simulink model "ANN_based_PI_Controlled_SAPF_pq_theory"  (R2023b)
settings: Solver=ode45  StartTime=0.0  StopTime=5  RelTol=1e-3  EnableMultiTasking=on
model workspace (MAT data in the model file):
  Ki = 1
  Kp = 0.1
libraries: spsDiodeLib x6, spsSeriesRLCBranchLib x5, spsCurrentMeasurementLib x4, spsThreePhaseBreakerLib x3, spsThreePhaseVIMeasurementLib x3, spsVoltageMeasurementLib x2, spsThreePhaseSeriesRLCBranchLib x2, spsThreePhaseSourceLib x1, simulink x1, dspfdesign x1, spsUniversalBridgeLib x1, sps_lib x1
settings Model: Creator=Jawad  LastModifiedBy=khana
settings SolverCC: AlgebraicLoopSolver=TrustRegion
settings DataIOCC: LimitDataPoints=on  SaveFormat=Array  SignalLoggingSaveFormat=ModelDataLogs  ReturnWorkspaceOutputs=off
settings OptimizationCC: ExpressionDepthLimit=2147483647  LifeSpan=inf
settings DebuggingCC: UnderspecifiedInitializationDetection=Classic  MergeDetectMultiDrivingBlocksExec=none  SolverPrmCheckMsg=warning  FcnCallInpInsideContextMsg=warning  UnconnectedInputMsg=warning  UnconnectedOutputMsg=warning  UnconnectedLineMsg=warning  StateNameClashWarn=warning  SFUnexpectedBacktrackingDiag=warning  SFNoUnconditionalDefaultTransitionDiag=warning  SFExecutionAtInitializationDiag=none  ArithmeticOperatorsInVariantConditions=warning
settings HardwareCC: ProdBitPerPointer=32  ProdBitPerSizeT=32  ProdBitPerPtrDiffT=32  ProdLargestAtomicFloat=None  ProdIntDivRoundTo=Undefined  ProdEndianess=Unspecified  ProdWordSize=32  ProdHWDeviceType=32-bit Generic
settings ModelReferenceCC: PropagateSignalLabelsOutOfModel=off
settings SFSimCC: SimUseLocalCustomCode=off  SimParseCustomCode=off  CustomCodeUndefinedFunction=UseInterfaceOnly
settings RTWCC: RTWUseLocalCustomCode=off
settings CodeAppCC: StateflowObjectComments=on
settings GRTTargetCC: TargetLangStandard=C89/C90 (ANSI)  CombineOutputUpdateFcns=off  GRTInterface=on
settings ConfigComp: CovMetricSettings=dw  CovSaveCumulativeToWorkspaceVar=on  CovSaveSingleToWorkspaceVar=on  CovExternalEMLEnable=off

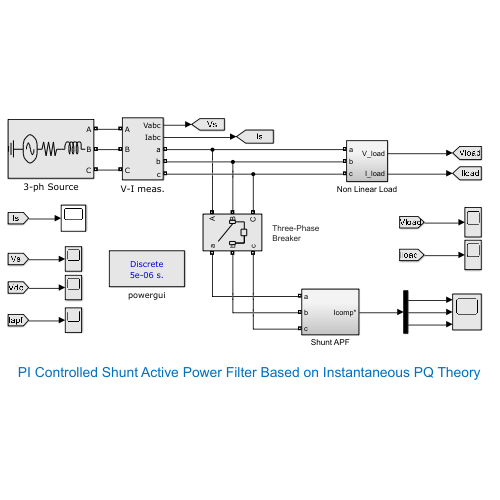
[thumbnail: Simulink's stored preview of the top-level diagram]
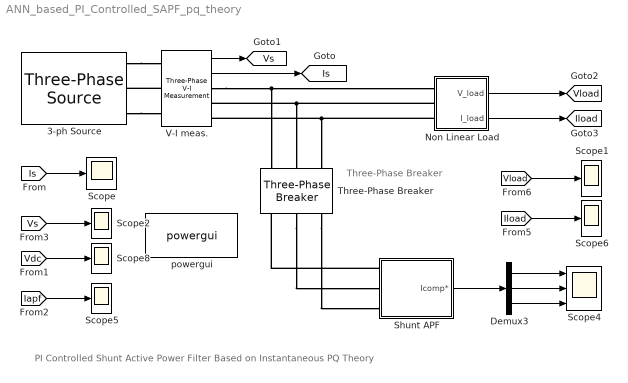
== system ANN_based_PI_Controlled_SAPF_pq_theory ==
  note: Three-Phase Breaker
  note: PI Controlled Shunt Active Power Filter Based on Instantaneous PQ Theory
  3-ph Source : spsThreePhaseSourceLib/Three-Phase Source  InternalConnection=Yg  VoltagePhases=off  Voltage=40  PhaseAngle=0  Voltage_phases=[25e3 25e3 25e3]/sqrt(3)  PhaseAngles_phases=[0 -120 +120]  Frequency=50  NonIdealSource=on  SpecifyImpedance=off  Resistance=0.001  Inductance=1e-8  ShortCircuitLevel=100e6  BaseVoltage=25e3  XRratio=7  BusType=swing  Pref=10e3  Qref=0  Prefabc=[10e3, 10e3, 10e3]  Qrefabc=[0, 0, 0]  Qmin=-inf  Qmax=inf
  Demux3 : Demux  Outputs=3
  Non Linear Load : Subsystem
  Scope{,1..2,5..6,8} (6 alike) : Scope
  Scope4 : Scope  NumInputPorts=3
  Shunt APF : Subsystem
  Three-Phase Breaker : spsThreePhaseBreakerLib/Three-Phase Breaker  InitialState=open  SwitchA=on  SwitchB=on  SwitchC=on  SwitchTimes=0.02  External=off  BreakerResistance=1e-6  SnubberResistance=1e6  SnubberCapacitance=inf  Measurements=None
  V-I meas. : spsThreePhaseVIMeasurementLib/Three-Phase V-I Measurement  VoltageMeasurement=phase-to-ground  SetLabelV=off  LabelV=Vabc  Vpu=off  VpuLL=off  CurrentMeasurement=yes  SetLabelI=off  LabelI=Iabc  Ipu=off  Pbase=100e6  Vbase=500e3  OutputType=Complex  PhasorSimulation=off  PSBequivalent=0
  powergui : sps_lib/powergui  Priority=1  SimulationMode=Discrete  SampleTime=5e-6  frequency=60  Iterations=50  frequencyindice=50  Pbase=100e6  ErrMax=1e-4  UnitsV=kV  UnitsW=MW  buscounter=0  FunctionMessages=off  echomessages=off  EnableUseOfTLC=off  CurrentSourceSwitches=off  DisableSnubberDevices=off  DisableRonSwitches=off  DisableVfSwitches=off  DisplayEquations=off  AutomaticDiscreteSolvers=off  SolverType=Tustin/Backward Euler (TBE)  Interpol=off  ExternalGateDelay=off  methode=off  Ts=100  x0status=blocks  SPID=off  SwTol=0  HookPort=off  NonlinearTolerance=1e-4  nMaxIteration=100  ContinueOnMaxIteration=off  RestoreLinks=warning  ResistiveCurrentMeasurement=off  Frange=[0:2:500]  Ylog=off  Xlog=on  ShowGrid=off  save=off  variable=ZData  structure=psb3phPWM1_str8  ZoomFFT=off  StartTime=0.035  cycles=2  DisplayStyle=2  fundamental=50  FreqAxis=off  MaxFrequency=10000  frequencyindicesteady=1  RmsSteady=1  display=off
  tag scope: Iload=global, Is=global, Vload=global, Vs=global
  wires:
  Non Linear Load/2(I_load) -> [Iload]
  V-I meas./1 -> [Vs]
  V-I meas./2 -> [Is]
  Demux3/1 -> Scope4/1
  Demux3/2 -> Scope4/2
  Demux3/3 -> Scope4/3
  Shunt APF/1(Icomp*) -> Demux3/1
  [Is] -> Scope/1
  [Vs] -> Scope2/1
  [Vdc] -> Scope8/1
  [Iapf] -> Scope5/1
  [Vload] -> Scope1/1
  [Iload] -> Scope6/1
  Non Linear Load/1(V_load) -> [Vload]
  connections:
  3-ph Source/RConn1 -- V-I meas./LConn1
  V-I meas./LConn2 -- 3-ph Source/RConn2
  3-ph Source/RConn3 -- V-I meas./LConn3
  V-I meas./RConn1 -- Three-Phase Breaker/LConn1 -- Non Linear Load/LConn1
  Non Linear Load/LConn2 -- Three-Phase Breaker/LConn2 -- V-I meas./RConn2
  Non Linear Load/LConn3 -- Three-Phase Breaker/LConn3 -- V-I meas./RConn3
  Shunt APF/LConn1 -- Three-Phase Breaker/RConn1
  Three-Phase Breaker/RConn2 -- Shunt APF/LConn2
  Three-Phase Breaker/RConn3 -- Shunt APF/LConn3

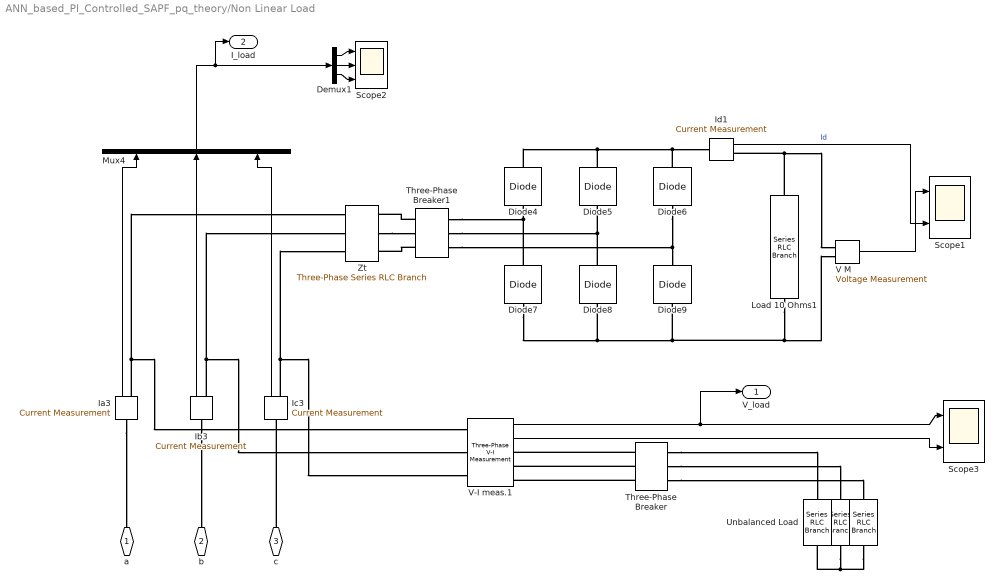
== system ANN_based_PI_Controlled_SAPF_pq_theory/Non Linear Load ==
  " " : spsSeriesRLCBranchLib/Series RLC Branch  LConnTagsString=__new0  RConnTagsString=__new0  BranchType=R  Resistance=4  Inductance=[]  SetiL0=off  InitialCurrent=0  Capacitance=[]  Setx0=off  InitialVoltage=0  Measurements=None
  "   " : spsSeriesRLCBranchLib/Series RLC Branch  LConnTagsString=__new0  RConnTagsString=__new0  BranchType=R  Resistance=6  Inductance=[]  SetiL0=off  InitialCurrent=0  Capacitance=[]  Setx0=off  InitialVoltage=0  Measurements=None
  Demux1 : Demux  Outputs=3
  Diode{4..9} (6 alike) : spsDiodeLib/Diode  Ron=1e-1  Lon=0  Vf=0.8  IC=0  UseSnubber=off  Rs=1000  Cs=0.1e-6  Measurements=off
      settings: AttributesFormatString=\n
  Ia3 : spsCurrentMeasurementLib/Current Measurement  PhasorSimulation=off  OutputType=Complex  PSBequivalent=0
  Ib3 : spsCurrentMeasurementLib/Current Measurement  PhasorSimulation=off  OutputType=Complex  PSBequivalent=0
  Ic3 : spsCurrentMeasurementLib/Current Measurement  PhasorSimulation=off  OutputType=Complex  PSBequivalent=0
  Id1 : spsCurrentMeasurementLib/Current Measurement  Tag=PoWeRsYsTeMmEaSuReMeNt  PhasorSimulation=off  OutputType=Magnitude  PSBequivalent=0
      settings: AttributesFormatString=\n
  Load 10 Ohms1 : spsSeriesRLCBranchLib/Series RLC Branch  LConnTagsString=__new0  RConnTagsString=__new0  BranchType=RL  Resistance=60  Inductance=10e-3  SetiL0=off  InitialCurrent=0  Capacitance=[]  Setx0=off  InitialVoltage=0  Measurements=None
  Mux4 : Mux  Inputs=3
  Scope1 : Scope  NumInputPorts=2
  Scope2 : Scope  NumInputPorts=3
  Scope3 : Scope  NumInputPorts=2
  Three-Phase Breaker : spsThreePhaseBreakerLib/Three-Phase Breaker  InitialState=open  SwitchA=on  SwitchB=on  SwitchC=on  SwitchTimes=0.2  External=off  BreakerResistance=1e-5  SnubberResistance=1e6  SnubberCapacitance=inf  Measurements=None
  Three-Phase Breaker1 : spsThreePhaseBreakerLib/Three-Phase Breaker  InitialState=open  SwitchA=on  SwitchB=on  SwitchC=on  SwitchTimes=0  External=off  BreakerResistance=1e-5  SnubberResistance=1e6  SnubberCapacitance=inf  Measurements=None
  Unbalanced Load : spsSeriesRLCBranchLib/Series RLC Branch  LConnTagsString=__new0  RConnTagsString=__new0  BranchType=R  Resistance=2  Inductance=[]  SetiL0=off  InitialCurrent=0  Capacitance=[]  Setx0=off  InitialVoltage=0  Measurements=None
  V M : spsVoltageMeasurementLib/Voltage Measurement  PhasorSimulation=off  OutputType=Complex  PSBequivalent=0
  V-I meas.1 : spsThreePhaseVIMeasurementLib/Three-Phase V-I Measurement  VoltageMeasurement=phase-to-ground  SetLabelV=off  LabelV=Vabc  Vpu=off  VpuLL=off  CurrentMeasurement=yes  SetLabelI=off  LabelI=Iabc  Ipu=off  Pbase=100e6  Vbase=500e3  OutputType=Complex  PhasorSimulation=off  PSBequivalent=0
  Zt : spsThreePhaseSeriesRLCBranchLib/Three-Phase Series RLC Branch  LConnTagsString=A|B|C  RConnTagsString=A|B|C  BranchType=RL  Resistance=0.01  Inductance=1e-3  Capacitance=1e-6  Measurements=None
  a : PMIOPort  Side=Left
  b : PMIOPort  Port=2  Side=Left
  c : PMIOPort  Port=3  Side=Left
  V_load : Outport
  I_load : Outport  Port=2
  wires:
  Mux4/1 -> I_load/1, Demux1/1
  Demux1/2 -> Scope2/2
  Demux1/3 -> Scope2/3
  Demux1/1 -> Scope2/1
  V M/1 -> Scope1/1
  Id1/1 -> Scope1/2  "Id"
  V-I meas.1/1 -> Scope3/1, V_load/1
  V-I meas.1/2 -> Scope3/2
  Ic3/1 -> Mux4/3
  Ib3/1 -> Mux4/2
  Ia3/1 -> Mux4/1
  connections:
  Ia3/LConn1 -- a/RConn1
  Ib3/LConn1 -- b/RConn1
  Ic3/RConn1 -- V-I meas.1/LConn3 -- Zt/LConn3
  Ib3/RConn1 -- V-I meas.1/LConn2 -- Zt/LConn2
  Ia3/RConn1 -- V-I meas.1/LConn1 -- Zt/LConn1
  Diode6/RConn1 -- Id1/LConn1 -- Diode4/RConn1 -- Diode5/RConn1
  Load 10 Ohms1/LConn1 -- Id1/RConn1 -- V M/LConn1
  Diode9/LConn1 -- Diode7/LConn1 -- Diode8/LConn1 -- V M/LConn2 -- Load 10 Ohms1/RConn1
  Unbalanced Load/RConn1 -- " "/RConn1 -- "   "/RConn1
  c/RConn1 -- Ic3/LConn1
  Three-Phase Breaker/LConn3 -- V-I meas.1/RConn3
  Three-Phase Breaker/LConn2 -- V-I meas.1/RConn2
  Three-Phase Breaker/LConn1 -- V-I meas.1/RConn1
  Three-Phase Breaker/RConn1 -- Unbalanced Load/LConn1
  Three-Phase Breaker/RConn2 -- " "/LConn1
  Three-Phase Breaker/RConn3 -- "   "/LConn1
  Diode7/RConn1 -- Three-Phase Breaker1/RConn1 -- Diode4/LConn1
  Diode8/RConn1 -- Three-Phase Breaker1/RConn2 -- Diode5/LConn1
  Diode6/LConn1 -- Diode9/RConn1 -- Three-Phase Breaker1/RConn3
  Three-Phase Breaker1/LConn1 -- Zt/RConn1
  Zt/RConn2 -- Three-Phase Breaker1/LConn2
  Three-Phase Breaker1/LConn3 -- Zt/RConn3

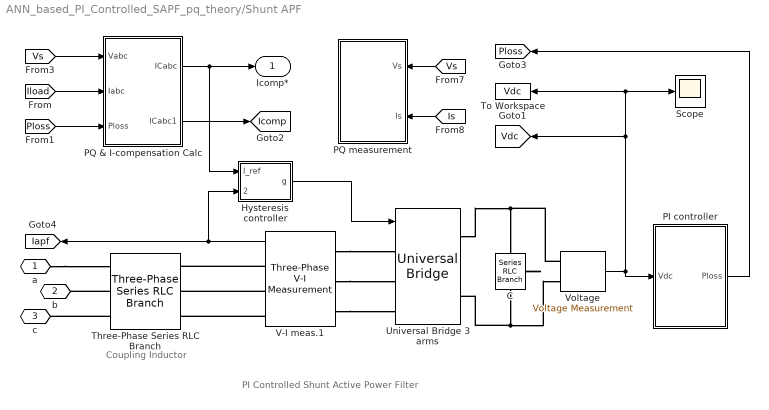
== system ANN_based_PI_Controlled_SAPF_pq_theory/Shunt APF ==
  note: Coupling Inductor
  note: PI Controlled Shunt Active Power Filter
  C : spsSeriesRLCBranchLib/Series RLC Branch  LConnTagsString=__new0  RConnTagsString=__new0  BranchType=C  Resistance=1  Inductance=1e-3  SetiL0=off  InitialCurrent=0  Capacitance=3.5e-6  Setx0=off  InitialVoltage=400  Measurements=None
  Hysteresis controller : Subsystem
  PI controller : Subsystem
  PQ & I-compensation Calc : Subsystem
  PQ measurement : Subsystem
  Scope : Scope
  Three-Phase Series RLC Branch : spsThreePhaseSeriesRLCBranchLib/Three-Phase Series RLC Branch  LConnTagsString=A|B|C  RConnTagsString=A|B|C  BranchType=L  Resistance=1e9  Inductance=10e-3  Capacitance=.2e-3  Measurements=None
  To Workspace : ToWorkspace  VariableName=Vdc  SaveFormat=Timeseries  SampleTime=-1
  Universal Bridge 3 arms : spsUniversalBridgeLib/Universal Bridge  Arms=3  SnubberResistance=10000  SnubberCapacitance=inf  Device=IGBT / Diodes  Ron=1e-4  Lon=0  ForwardVoltages="[  1  1  ]"  ForwardVoltage=.8  GTOparameters=[ 10e-6 , 20e-6 ]  IGBTparameters=[ 1e-6 , 2e-6 ]  Measurements=None  Measurements_2=None  converterType=Rectifier
      settings: AttributesFormatString=\n
  V-I meas.1 : spsThreePhaseVIMeasurementLib/Three-Phase V-I Measurement  VoltageMeasurement=phase-to-ground  SetLabelV=on  LabelV=Vnm  Vpu=off  VpuLL=off  CurrentMeasurement=yes  SetLabelI=off  LabelI=Iabc  Ipu=off  Pbase=100e6  Vbase=500e3  OutputType=Complex  PhasorSimulation=off  PSBequivalent=0
  Voltage : spsVoltageMeasurementLib/Voltage Measurement  PhasorSimulation=off  OutputType=Complex  PSBequivalent=0
  a : PMIOPort  Side=Left
  b : PMIOPort  Port=2  Side=Left
  c : PMIOPort  Port=3  Side=Left
  Icomp* : Outport
  tag scope: Iapf=global, Icomp=global, Ploss=global, Vdc=global
  wires:
  [Iload] -> PQ & I-compensation Calc/2(Iabc)
  V-I meas.1/1 -> [Iapf], Hysteresis controller/2(I_meas)
  Hysteresis controller/1(g) -> Universal Bridge 3 arms/1
  PQ & I-compensation Calc/1(ICabc) -> Icomp*/1, Hysteresis controller/1(I_ref)
  Voltage/1 -> To Workspace/1, Scope/1, [Vdc], PI controller/1(Vdc)
  [Vs] -> PQ & I-compensation Calc/1(Vabc)
  PQ & I-compensation Calc/2(ICabc1) -> [Icomp]
  PI controller/1(Ploss) -> [Ploss]
  [Ploss] -> PQ & I-compensation Calc/3(Ploss)
  [Vs] -> PQ measurement/1(Vs)
  [Is] -> PQ measurement/2(Is)
  connections:
  Voltage/LConn1 -- C/LConn1 -- Universal Bridge 3 arms/RConn1
  V-I meas.1/LConn1 -- Universal Bridge 3 arms/LConn1
  V-I meas.1/LConn2 -- Universal Bridge 3 arms/LConn2
  V-I meas.1/RConn3 -- Three-Phase Series RLC Branch/LConn3
  V-I meas.1/RConn2 -- Three-Phase Series RLC Branch/LConn2
  V-I meas.1/LConn3 -- Universal Bridge 3 arms/LConn3
  V-I meas.1/RConn1 -- Three-Phase Series RLC Branch/LConn1
  a/RConn1 -- Three-Phase Series RLC Branch/RConn1
  Three-Phase Series RLC Branch/RConn2 -- b/RConn1
  Three-Phase Series RLC Branch/RConn3 -- c/RConn1
  C/RConn1 -- Voltage/LConn2 -- Universal Bridge 3 arms/RConn2

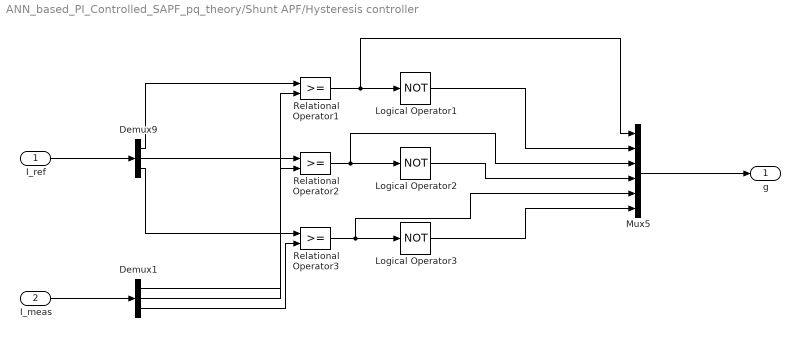
== system ANN_based_PI_Controlled_SAPF_pq_theory/Shunt APF/Hysteresis controller ==
  I_ref : Inport
  I_meas : Inport  Port=2
  Demux1 : Demux  Outputs=3
  Demux9 : Demux  Outputs=3
  Logical Operator1 : Logic  Operator=NOT  AllPortsSameDT=off  OutDataTypeStr=boolean
  Logical Operator2 : Logic  Operator=NOT  AllPortsSameDT=off  OutDataTypeStr=boolean
  Logical Operator3 : Logic  Operator=NOT  AllPortsSameDT=off  OutDataTypeStr=boolean
  Mux5 : Mux  Inputs=6
  Relational Operator1 : RelationalOperator  OutDataTypeStr=boolean  ZeroCross=off  InputSameDT=off
  Relational Operator2 : RelationalOperator  OutDataTypeStr=boolean  ZeroCross=off  InputSameDT=off
  Relational Operator3 : RelationalOperator  OutDataTypeStr=boolean  ZeroCross=off  InputSameDT=off
  g : Outport
  wires:
  Relational Operator1/1 -> Logical Operator1/1, Mux5/1
  Relational Operator2/1 -> Logical Operator2/1, Mux5/3
  Relational Operator3/1 -> Logical Operator3/1, Mux5/5
  Demux9/1 -> Relational Operator1/1
  Demux9/3 -> Relational Operator3/1
  Logical Operator1/1 -> Mux5/2
  Logical Operator2/1 -> Mux5/4
  Logical Operator3/1 -> Mux5/6
  Mux5/1 -> g/1
  Demux9/2 -> Relational Operator2/1
  Demux1/1 -> Relational Operator1/2
  Demux1/2 -> Relational Operator2/2
  Demux1/3 -> Relational Operator3/2
  I_ref/1 -> Demux9/1
  I_meas/1 -> Demux1/1

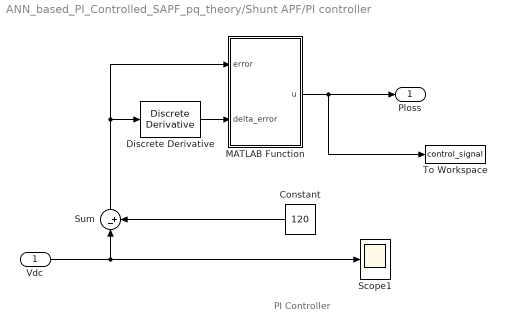
== system ANN_based_PI_Controlled_SAPF_pq_theory/Shunt APF/PI controller ==
  note: PI Controller
  Vdc : Inport
  Constant : Constant  Value=120
  Discrete Derivative : simulink/Discrete/Discrete Derivative  gainval=1.0  ICPrevScaledInput=0.0  OutMin=[]  OutMax=[]  OutDataType=fixdt(1, 16)  OutScaling=2^-10  DoSatur=off
  MATLAB Function : MATLAB Function  TreatAsAtomicUnit=on
  Scope1 : Scope
  Sum : Sum  Inputs=|-+
  To Workspace : ToWorkspace  VariableName=control_signal  SaveFormat=Timeseries  SampleTime=-1
  Ploss : Outport
  wires:
  Constant/1 -> Sum/2
  Sum/1 -> MATLAB Function/1(error), Discrete Derivative/1
  MATLAB Function/1(u) -> Ploss/1, To Workspace/1
  Vdc/1 -> Scope1/1, Sum/1
  Discrete Derivative/1 -> MATLAB Function/2(delta_error)

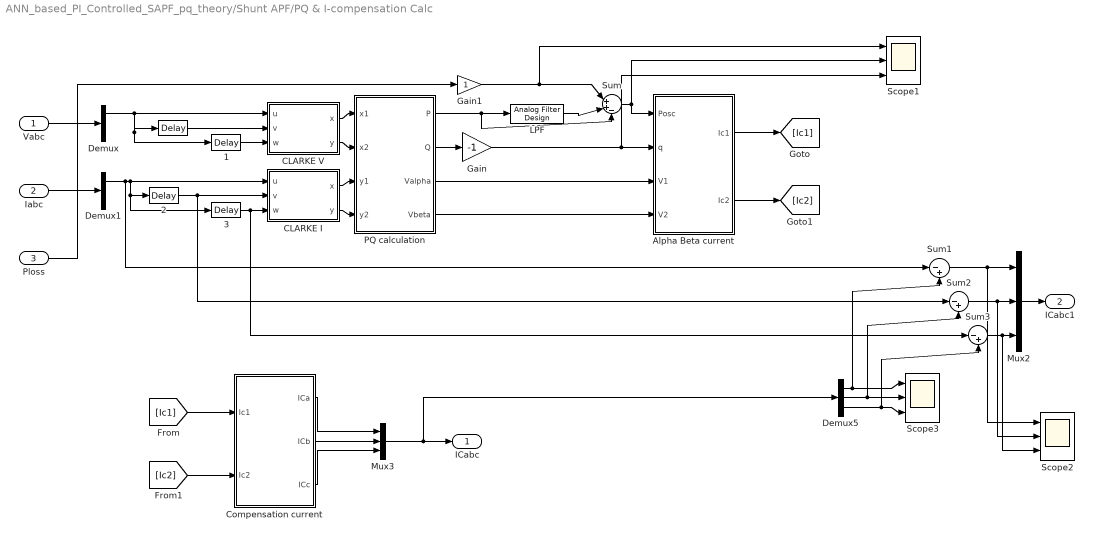
== system ANN_based_PI_Controlled_SAPF_pq_theory/Shunt APF/PQ & I-compensation Calc ==
  Vabc : Inport
  Iabc : Inport  Port=2
  Ploss : Inport  Port=3
  " " : TransportDelay  DelayTime=0.006666666
  " 1" : TransportDelay  DelayTime=0.013333333
  " 2" : TransportDelay  DelayTime=0.006666666
  " 3" : TransportDelay  DelayTime=0.013333333
  Alpha Beta current : MATLAB Function  TreatAsAtomicUnit=on
  CLARKE I : MATLAB Function  TreatAsAtomicUnit=on
  CLARKE V : MATLAB Function  TreatAsAtomicUnit=on
  Compensation current : MATLAB Function  TreatAsAtomicUnit=on
  Demux : Demux  Outputs=3
  Demux1 : Demux  Outputs=3
  Demux5 : Demux  Outputs=3
  Gain : Gain  Gain=-1
  Gain1 : Gain
  LPF : dspfdesign/Analog Filter Design  method=Butterworth  filttype=Lowpass  N=5  Wlo=2*pi*50  Whi=80  Rp=2  Rs=40
  Mux2 : Mux  Inputs=3
  Mux3 : Mux  Inputs=3
  PQ calculation : MATLAB Function  TreatAsAtomicUnit=on
  Scope1 : Scope  NumInputPorts=3
  Scope2 : Scope  NumInputPorts=3
  Scope3 : Scope  NumInputPorts=3
  Sum : Sum  Inputs=|++-
  Sum1 : Sum  Inputs=|-+
  Sum2 : Sum  Inputs=|-+
  Sum3 : Sum  Inputs=|-+
  ICabc : Outport
  ICabc1 : Outport  Port=2
  wires:
  Iabc/1 -> Demux1/1
  Vabc/1 -> Demux/1
  [Ic1] -> Compensation current/1(Ic1)
  [Ic2] -> Compensation current/2(Ic2)
  Compensation current/1(ICa) -> Mux3/1
  Compensation current/2(ICb) -> Mux3/2
  Compensation current/3(ICc) -> Mux3/3
  CLARKE V/1(x) -> PQ calculation/1(x1)
  CLARKE V/2(y) -> PQ calculation/2(x2)
  CLARKE I/1(x) -> PQ calculation/3(y1)
  PQ calculation/2(Q) -> Gain/1
  PQ calculation/1(P) -> LPF/1, Sum/3
  Gain/1 -> Alpha Beta current/2(q), Scope1/3
  PQ calculation/3(Valpha) -> Alpha Beta current/3(V1)
  Alpha Beta current/1(Ic1) -> [Ic1]
  Alpha Beta current/2(Ic2) -> [Ic2]
  CLARKE I/2(y) -> PQ calculation/4(y2)
  PQ calculation/4(Vbeta) -> Alpha Beta current/4(V2)
  Demux/1 -> " "/1, " 1"/1, CLARKE V/1(u)
  Demux1/1 -> Sum1/1, CLARKE I/1(u), " 3"/1, " 2"/1
  LPF/1 -> Sum/2
  Sum/1 -> Alpha Beta current/1(Posc), Scope1/2
  Gain1/1 -> Sum/1, Scope1/1
  Mux3/1 -> ICabc/1, Demux5/1
  Demux5/1 -> Scope3/1, Sum1/2
  Demux5/2 -> Scope3/2, Sum2/2
  Demux5/3 -> Scope3/3, Sum3/2
  Ploss/1 -> Gain1/1
  Sum1/1 -> Mux2/1, Scope2/1
  Sum2/1 -> Mux2/2, Scope2/2
  Sum3/1 -> Mux2/3, Scope2/3
  Mux2/1 -> ICabc1/1
  " "/1 -> CLARKE V/2(v)
  " 1"/1 -> CLARKE V/3(w)
  " 2"/1 -> CLARKE I/2(v), Sum2/1
  " 3"/1 -> CLARKE I/3(w), Sum3/1

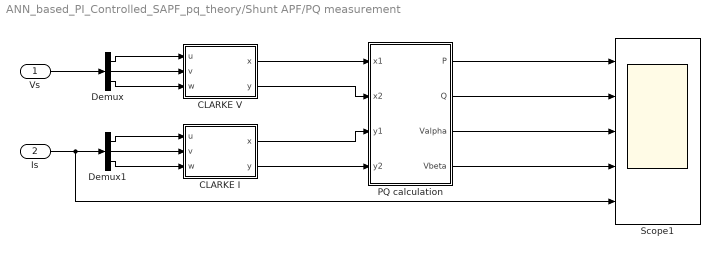
== system ANN_based_PI_Controlled_SAPF_pq_theory/Shunt APF/PQ measurement ==
  Vs : Inport
  Is : Inport  Port=2
  CLARKE I : MATLAB Function  TreatAsAtomicUnit=on
  CLARKE V : MATLAB Function  TreatAsAtomicUnit=on
  Demux : Demux  Outputs=3
  Demux1 : Demux  Outputs=3
  PQ calculation : MATLAB Function  TreatAsAtomicUnit=on
  Scope1 : Scope  NumInputPorts=5
  wires:
  CLARKE V/1(x) -> PQ calculation/1(x1)
  CLARKE V/2(y) -> PQ calculation/2(x2)
  CLARKE I/1(x) -> PQ calculation/3(y1)
  CLARKE I/2(y) -> PQ calculation/4(y2)
  Demux/1 -> CLARKE V/1(u)
  Demux/2 -> CLARKE V/2(v)
  Demux/3 -> CLARKE V/3(w)
  Demux1/1 -> CLARKE I/1(u)
  Demux1/2 -> CLARKE I/2(v)
  Demux1/3 -> CLARKE I/3(w)
  Vs/1 -> Demux/1
  Is/1 -> Demux1/1, Scope1/5
  PQ calculation/1(P) -> Scope1/1
  PQ calculation/2(Q) -> Scope1/2
  PQ calculation/3(Valpha) -> Scope1/3
  PQ calculation/4(Vbeta) -> Scope1/4

== matlab function ANN_based_PI_Controlled_SAPF_pq_theory/Shunt APF/PI controller/MATLAB Function ==
  data: error input; u output; delta_error input
function u = fcn(error, delta_error)
    u = nn_controller_pso(error, delta_error);
end

== matlab function ANN_based_PI_Controlled_SAPF_pq_theory/Shunt APF/PQ & I-compensation Calc/CLARKE I ==
  data: u input; x output; v input; w input; y output
function [x,y] = ICT(u,v,w)
%#em1

x = sqrt(2/3)*(u-(0.5*v)-(0.5*w));
y = sqrt(2)*(0+(0.5*v)-(0.5*w));

== matlab function ANN_based_PI_Controlled_SAPF_pq_theory/Shunt APF/PQ & I-compensation Calc/CLARKE V ==
  data: u input; x output; v input; w input; y output
function [x,y] = VCT(u,v,w)
%#em1

x = sqrt(2/3)*(u-(0.5*v)-(0.5*w));
y = sqrt(2)*(0+(0.5*v)-(0.5*w));

== matlab function ANN_based_PI_Controlled_SAPF_pq_theory/Shunt APF/PQ & I-compensation Calc/PQ calculation ==
  data: x1 input; P output; Q output; x2 input; y1 input; y2 input; Valpha output; Vbeta output
function [P,Q,Valpha,Vbeta] = PQ(x1,x2,y1,y2)
%#em1

P = (x1*y1)+(x2*y2);
Q = (x2*y1)-(x1*y2);
Valpha = x1;
Vbeta = x2;

== matlab function ANN_based_PI_Controlled_SAPF_pq_theory/Shunt APF/PQ & I-compensation Calc/Compensation current ==
  data: Ic1 input; ICa output; Ic2 input; ICb output; ICc output
function [ICa,ICb,ICc] = Ical(Ic1,Ic2)
%#em1

ICa = sqrt(2/3)*(Ic1);
ICb = sqrt(2/3)*((-0.5*Ic1)+((sqrt(3)/2)*Ic2));
ICc = sqrt(2/3)*((-0.5*Ic1)-((sqrt(3)/2)*Ic2));

== matlab function ANN_based_PI_Controlled_SAPF_pq_theory/Shunt APF/PQ & I-compensation Calc/Alpha Beta current ==
  data: Posc input; Ic1 output; q input; V1 input; Ic2 output; V2 input
function [Ic1,Ic2] = ICOM(Posc,q,V1,V2)
%#em1

Ic1 = (-1/(V1^2 + V2^2))*((Posc*V1)+(q*V2));
Ic2 = (-1/(V1^2 + V2^2))*((Posc*V2)-(q*V1));

== matlab function ANN_based_PI_Controlled_SAPF_pq_theory/Shunt APF/PQ measurement/CLARKE I ==
  data: u input; x output; v input; w input; y output
function [x,y] = ICT(u,v,w)
%#em1

x = sqrt(2/3)*(u-(0.5*v)-(0.5*w));
y = sqrt(2)*(0+(0.5*v)-(0.5*w));

== matlab function ANN_based_PI_Controlled_SAPF_pq_theory/Shunt APF/PQ measurement/CLARKE V ==
  data: u input; x output; v input; w input; y output
function [x,y] = VCT(u,v,w)
%#em1

x = sqrt(2/3)*(u-(0.5*v)-(0.5*w));
y = sqrt(2)*(0+(0.5*v)-(0.5*w));

== matlab function ANN_based_PI_Controlled_SAPF_pq_theory/Shunt APF/PQ measurement/PQ calculation ==
  data: x1 input; P output; Q output; x2 input; y1 input; y2 input; Valpha output; Vbeta output
function [P,Q,Valpha,Vbeta] = PQ(x1,x2,y1,y2)
%#em1

P = (x1*y1)+(x2*y2);
Q = (x2*y1)-(x1*y2);
Valpha = x1;
Vbeta = x2;
